simulink library "raspi_drivers"  (R2018b)
settings: Solver=VariableStepAuto  StartTime=0.0  StopTime=10.0  RelTol=1e-3
InitFcn:
  | Ts = 1/50;
undefined symbols (not defined in the file): H
settings Model: Creator=marti  LastModifiedBy=marti
settings SFSimCC: SimUseLocalCustomCode=off
settings RTWCC: RTWUseLocalCustomCode=off
settings CodeAppCC: StateflowObjectComments=on

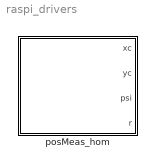
== system raspi_drivers ==
  posMeas_hom : Subsystem  InitFcn=|  mask{H=H}
      | %simul_time = str2num(get_param(gcs, 'StopTime'));
      | %fps = 50;
      | %num_frames = round(50*(simul_time+30));
      | %stream = 0;
      | %exposition_time = 5;
      | 
      | %if ~exist('mypi')
      | % mypi = raspi(ip_rpi, rpi_user, rpi_passwd);
      | %end
      | % run the script measuring the position on raspi
      | %rpi_posMes_run( mypi, fps, num_frames, stream, exposition_time )
      mask prompts: H "Calibration Matrix"

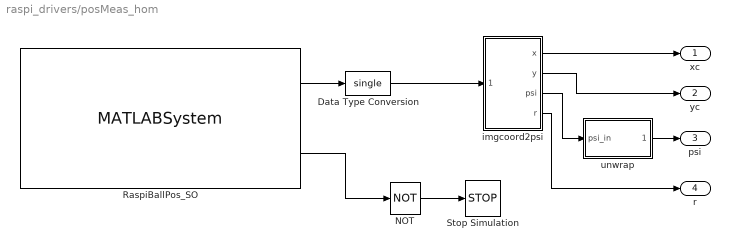
== system raspi_drivers/posMeas_hom ==
  Data Type Conversion : DataTypeConversion  OutDataTypeStr=single
  NOT : Logic  Operator=NOT  IconShape=distinctive  AllPortsSameDT=off  OutDataTypeStr=boolean
  RaspiBallPos_SO : MATLABSystem  System=RaspiBallPos  shm_key=3145914  framerate=50  N=1000  objects=1  km=H  notfound=nan  execScript=off  concatenateOutputs=off  rotation=off  found_output=on
      mask Type: RaspiBallPos
      mask Display:
      | disp('RaspiBallPos');
      | port_label('output',1,'Position 1 [x;y]');
      | port_label('output',2,'Object found?');
  Stop Simulation : Stop
  imgcoord2psi : Subsystem
  unwrap : Subsystem
  xc : Outport
  yc : Outport  Port=2
  psi : Outport  Port=3
  r : Outport  Port=4
  wires:
  RaspiBallPos_SO/1 -> Data Type Conversion/1
  imgcoord2psi/3(psi) -> unwrap/1(psi_in)
  unwrap/1(psi_out) -> psi/1
  imgcoord2psi/1(x) -> xc/1
  imgcoord2psi/2(y) -> yc/1
  imgcoord2psi/4(r) -> r/1
  RaspiBallPos_SO/2 -> NOT/1
  NOT/1 -> Stop Simulation/1
  Data Type Conversion/1 -> imgcoord2psi/1(xy_img)

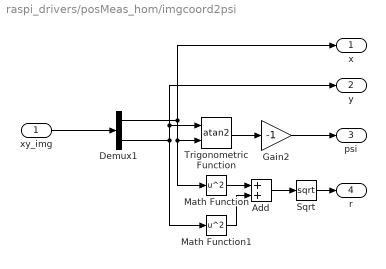
== system raspi_drivers/posMeas_hom/imgcoord2psi ==
  xy_img : Inport
  Add : Sum
  Demux1 : Demux  Outputs=2
  Gain2 : Gain  Gain=-1  OutDataTypeStr=single
  Math Function : Math  Operator=square  SaturateOnIntegerOverflow=on
  Math Function1 : Math  Operator=square  SaturateOnIntegerOverflow=on
  Sqrt : Sqrt  SaturateOnIntegerOverflow=on
  Trigonometric Function : Trigonometry  Operator=atan2  OutputSignalType=real
  x : Outport
  y : Outport  Port=2
  psi : Outport  Port=3
  r : Outport  Port=4
  wires:
  Demux1/2 -> y/1, Trigonometric Function/1, Math Function1/1
  xy_img/1 -> Demux1/1
  Demux1/1 -> x/1, Math Function/1, Trigonometric Function/2
  Trigonometric Function/1 -> Gain2/1
  Gain2/1 -> psi/1
  Add/1 -> Sqrt/1
  Math Function/1 -> Add/1
  Math Function1/1 -> Add/2
  Sqrt/1 -> r/1

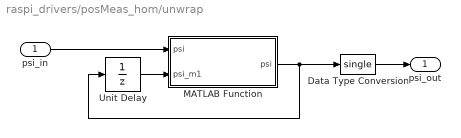
== system raspi_drivers/posMeas_hom/unwrap ==
  psi_in : Inport
  Data Type Conversion : DataTypeConversion  OutDataTypeStr=single
  MATLAB Function : MATLAB Function  TreatAsAtomicUnit=on
  Unit Delay : UnitDelay  InitialCondition=single(0)  SampleTime=-1
  psi_out : Outport
  wires:
  MATLAB Function/1(psi) -> Data Type Conversion/1, Unit Delay/1
  Unit Delay/1 -> MATLAB Function/2(psi_m1)
  psi_in/1 -> MATLAB Function/1("psi ")
  Data Type Conversion/1 -> psi_out/1

== matlab function raspi_drivers/posMeas_hom/unwrap/MATLAB Function ==
  data: psi input; psi output; psi_m1 input
function psi = unwrap(psi, psi_m1)
%%% The code is taken from the Matlab function unwrap

% Unwrap phase angles.  Algorithm minimizes the incremental phase variation 
% by constraining it to the range [-pi,pi]
dp = psi - psi_m1;                % Incremental phase variations

% Compute an integer describing how many times 2*pi we are off:
% dp in [-pi, pi]: dp_corr = 0,
% elseif dp in [-3*pi, 3*pi]: dp_corr = 1,
% else if dp in [-5*pi, 5*pi]: dp_corr = 2, ...
dp_corr = dp./(2*pi);

% We want to do round(dp_corr), except that we want the tie-break at n+0.5
% to round towards zero instead of away from zero (that is, (2n+1)*pi will
% be shifted by 2n*pi, not by (2n+2)*pi):
roundDown = abs(rem(dp_corr, 1)) <= 0.5;
dp_corr(roundDown) = fix(dp_corr(roundDown));

dp_corr = round(dp_corr);

% Stop the jump from happening if dp < cutoff (no effect if cutoff <= pi)
dp_corr(abs(dp) < pi) = 0;

% Integrate corrections and add to P to produce smoothed phase values
psi = single(psi - (2*pi)*cumsum(dp_corr,1));
